simulink model "sim_topic3"  (R2023b)
settings: Solver=FixedStepAuto  StartTime=0.0  StopTime=T_sim  FixedStep=dt_sim  RelTol=1e-3
undefined symbols (not defined in the file): den_Gd_tf_1, den_Gp_tf, num_Gd_tf_1, num_Gp_tf, T
settings Model: Creator=user  LastModifiedBy=user

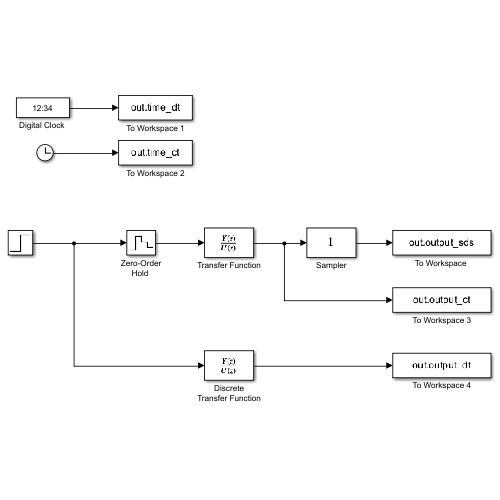
[thumbnail: Simulink's stored preview of the top-level diagram]
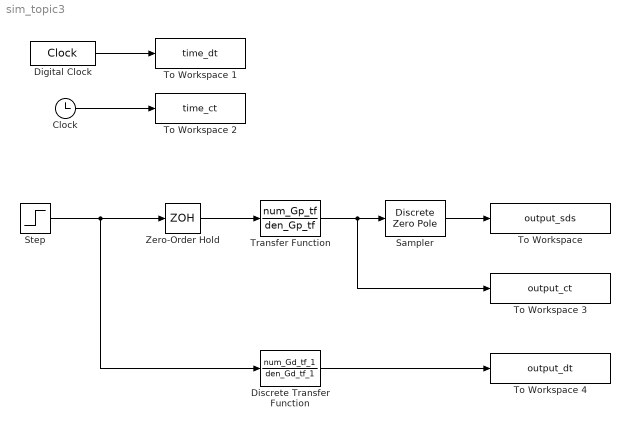
== system sim_topic3 ==
  Clock : Clock
  "Digital Clock " : DigitalClock  SampleTime=T
  Discrete Transfer Function : DiscreteTransferFcn  Numerator=num_Gd_tf_1  Denominator=den_Gd_tf_1
  Sampler : DiscreteZeroPole  Zeros=[]  Poles=[]  Gain=1  SampleTime=T
  Step : Step  Time=0  SampleTime=T
  "To Workspace " : ToWorkspace  VariableName=output_sds  SampleTime=T
  To Workspace 1 : ToWorkspace  VariableName=time_dt  SampleTime=T
  To Workspace 2 : ToWorkspace  VariableName=time_ct  SampleTime=-1
  To Workspace 3 : ToWorkspace  VariableName=output_ct  SampleTime=-1
  To Workspace 4 : ToWorkspace  VariableName=output_dt  SampleTime=T
  Transfer Function : TransferFcn  Numerator=num_Gp_tf  Denominator=den_Gp_tf
  "Zero-Order Hold " : ZeroOrderHold  SampleTime=-1
  wires:
  Step/1 -> Discrete Transfer Function/1, "Zero-Order Hold "/1
  Clock/1 -> To Workspace 2/1
  "Zero-Order Hold "/1 -> Transfer Function/1
  "Digital Clock "/1 -> To Workspace 1/1
  Sampler/1 -> "To Workspace "/1
  Discrete Transfer Function/1 -> To Workspace 4/1
  Transfer Function/1 -> To Workspace 3/1, Sampler/1
